simulink model "robotsimulation_grav"  (R2021a)
settings: Solver=VariableStepAuto  StartTime=0.0  StopTime=5  FixedStep=1e-2  RelTol=1e-3
values from neighbouring files (symbols this model uses):
  fext = zeros(6,8)    [simIRB120.m]    (also in simIRB120_S.m; simIRB120_f.m; simIRB120_grav.m; simIRB120_lin.m)
  kd = [2.5;2.5;1;5;5;5]    [simIRB120.m]    (also in simIRB120_S.m = [2.5;4.5;2;.1;.1;.1]; simIRB120_f.m; simIRB120_grav.m = [2.5;4.5;2;.1;.1;.1]; simIRB120_lin.m = [3;3;3;5;5;5])
  ki = [.1;.1;.1;0;0;0]    [simIRB120.m]    (also in simIRB120_S.m; simIRB120_f.m; simIRB120_grav.m; simIRB120_lin.m = [.1;.5;.2;.1;.1;.1])
  kp = [1.5;1.5;1.5;.1;.1;.1]    [simIRB120.m]    (also in simIRB120_S.m = [1.5;1.5;1.5;1;1;1]; simIRB120_f.m; simIRB120_grav.m = [1.5;1.5;1.5;1;1;1]; simIRB120_lin.m = [5;5;5;5;5;5])
  qdes = (rand(6,1)-.5)*2*pi    [simIRB120.m]    (also in simIRB120_S.m = q7(:,i); simIRB120_f.m; simIRB120_grav.m; simIRB120_lin.m = [0;pi/2;-pi/2;0;0;0])
  qdotinit = zeros(6,1)    [simIRB120.m]    (also in simIRB120_S.m = simout.qdot(end,:); simIRB120_f.m; simIRB120_grav.m; simIRB120_lin.m)
  qinit = zeros(6,1)    [simIRB120.m]    (also in simIRB120_S.m = simout.q(end,:); simIRB120_f.m; simIRB120_grav.m; simIRB120_lin.m)
  tau_zeros = zeros(6,1)    [simIRB120.m]    (also in simIRB120_S.m; simIRB120_f.m; simIRB120_grav.m; simIRB120_lin.m)
libraries: robotmaniplib x1, pid_lib x1
settings Model: Creator=wen  LastModifiedBy=frazic
settings SolverCC: AlgebraicLoopSolver=TrustRegion
settings DebuggingCC: SFMachineParentedDataDiag=warning

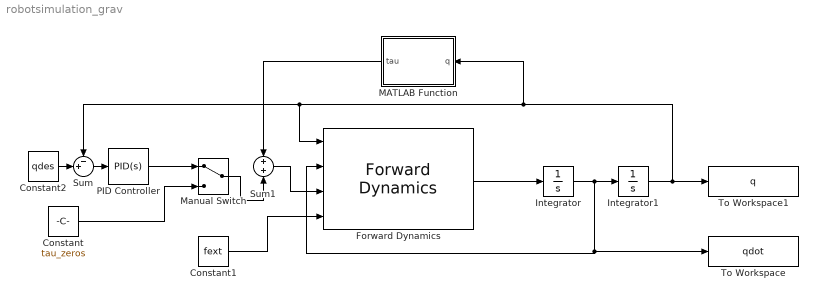
== system robotsimulation_grav ==
  Constant : Constant  Value=tau_zeros
  Constant1 : Constant  Value=fext
  Constant2 : Constant  Value=qdes
  Forward Dynamics : robotmaniplib/Forward Dynamics  RigidBodyTree=abb  SimulateUsing=Interpreted execution
  Integrator : Integrator  InitialCondition=qdotinit
  Integrator1 : Integrator  InitialCondition=qinit
  MATLAB Function : MATLAB Function  TreatAsAtomicUnit=on
  Manual Switch : ManualSwitch
  PID Controller : pid_lib/PID Controller  Controller=PID  Form=Parallel  TimeDomain=Continuous-time  UseExternalTs=off  SampleTime=-1  IntegratorMethod=Forward Euler  FilterMethod=Forward Euler  ControllerParametersSource=internal  P=kp  I=ki  D=kd  UseFilter=on  N=100  TunerSelectOption=Transfer Function Based (PID Tuner App)  InitialConditionSource=internal  InitialConditionForIntegrator=0  InitialConditionForFilter=0  DifferentiatorICPrevScaledInput=0  ExternalReset=none  TrackingMode=off  Kt=1  LimitOutput=off  SatLimitsSource=internal  UpperSaturationLimit=inf  LowerSaturationLimit=-inf  LinearizeAsGain=on  AntiWindupMode=none  Kb=1  POutMin=[]  POutMax=[]  IOutMin=[]  IOutMax=[]  DOutMin=[]  DOutMax=[]  NOutMin=[]  NOutMax=[]  SumOutMin=[]  SumOutMax=[]  SaturationOutMin=[]  SaturationOutMax=[]  PParamMin=[]  PParamMax=[]  IParamMin=[]  IParamMax=[]  DParamMin=[]  DParamMax=[]  NParamMin=[]  NParamMax=[]  KbParamMin=[]  KbParamMax=[]  KtParamMin=[]  KtParamMax=[]  KbOutMin=[]  KbOutMax=[]  KtOutMin=[]  KtOutMax=[]  IntegratorOutMin=[]  IntegratorOutMax=[]  FilterOutMin=[]  FilterOutMax=[]  SumI1OutMin=[]  SumI1OutMax=[]  SumI2OutMin=[]  SumI2OutMax=[]  SumI3OutMin=[]  SumI3OutMax=[]  SumI4OutMin=[]  SumI4OutMax=[]  SumDOutMin=[]  SumDOutMax=[]  DifferentiatorOutMin=[]  DifferentiatorOutMax=[]  FilterDiffOutCoefMin=[]  FilterDiffOutCoefMax=[]  ReciprocalOutMin=[]  ReciprocalOutMax=[]  SumDenOutMin=[]  SumDenOutMax=[]  SumNumOutMin=[]  SumNumOutMax=[]  DivideOutMin=[]  DivideOutMax=[]  UdiffTsProdOutMin=[]  UdiffTsProdOutMax=[]  NTsProdOutMin=[]  NTsProdOutMax=[]  UintegralTsProdOutMin=[]  UintegralTsProdOutMax=[]  UngainTsProdOutMin=[]  UngainTsProdOutMax=[]  IntegratorContinuousStateAttributes=''  IntegratorStateMustResolveToSignalObject=off  IntegratorRTWStateStorageClass=Auto  FilterContinuousStateAttributes=''  FilterStateMustResolveToSignalObject=off  FilterRTWStateStorageClass=Auto  ParallelPVariant=InternalParameters  IdealPVariant=Disabled  IVariant=InternalParameters  DVariant=InternalParameters  IntegratorVariant=Continuous  SatVariant=Disabled  AWVariant=Passthrough  PCopyVariant=Disabled  TRVariant=Disabled  FdbkBlocksVariant=Forward  IdealPFdbkVariant=Disabled  SatFdbkVariant=Disabled  DerivativeFilterVariant=ContFilter  NVariant=InternalParameters  NCopyVariant=Disabled  FilterICVariant=InternalICsFilter  IntegratorICVariant=InternalICs  ExternalResetVariant=Disabled  TRSumVariant=Passthrough  SumFdbkVariant=Disabled  SumVariant=Sum_PID  TsampFilterVariant=InternalTs  TsampNgainVariant=Passthrough  TsampIntegralVariant=Passthrough  ExternalSaturationOutDataTypeStr=Inherit: Same as second input
  Sum : Sum  Inputs=-+|
  Sum1 : Sum
  To Workspace : ToWorkspace  VariableName=qdot  SampleTime=-1
  To Workspace1 : ToWorkspace  VariableName=q  SampleTime=-1
  wires:
  Forward Dynamics/1 -> Integrator/1
  Integrator1/1 -> MATLAB Function/1(q), Sum/1, Forward Dynamics/1, To Workspace1/1
  PID Controller/1 -> Manual Switch/1
  Constant1/1 -> Forward Dynamics/4
  Sum/1 -> PID Controller/1
  Constant2/1 -> Sum/2
  Manual Switch/1 -> Sum1/2
  Constant/1 -> Manual Switch/2
  Integrator/1 -> Forward Dynamics/2, To Workspace/1, Integrator1/1
  MATLAB Function/1(tau) -> Sum1/1
  Sum1/1 -> Forward Dynamics/3

== matlab function robotsimulation_grav/MATLAB Function ==
  data: q input; tau output
function tau = Grav(q)
A=zeros(6,12);
A(2,1:5)=[sin(q(2)),sin(q(2)+q(3)),cos(q(2)+q(3)),sin(q(2)+q(3))*cos(q(4))*sin(q(5)),cos(q(2)+q(3))*cos(q(5))];
A(3,6:9)=[sin(q(2)+q(3)),cos(q(2)+q(3)),sin(q(2)+q(3))*cos(q(4))*sin(q(5)),cos(q(2)+q(3))*cos(q(5))];
A(4,10)=cos(q(2)+q(3))*sin(q(4))*sin(q(5));
A(5,11:12)=[sin(q(2)+q(3))*sin(q(5)),cos(q(2)+q(3))*cos(q(4))*cos(q(5))];
X=load('x_sol.mat');
tau = A*X.x;
